simulink model "Overflow"  (R2017b)
settings: Solver=VariableStepAuto  StartTime=0.0  StopTime=10.0  RelTol=1e-3
settings Model: Creator=MrGoshak  LastModifiedBy=MrGoshak

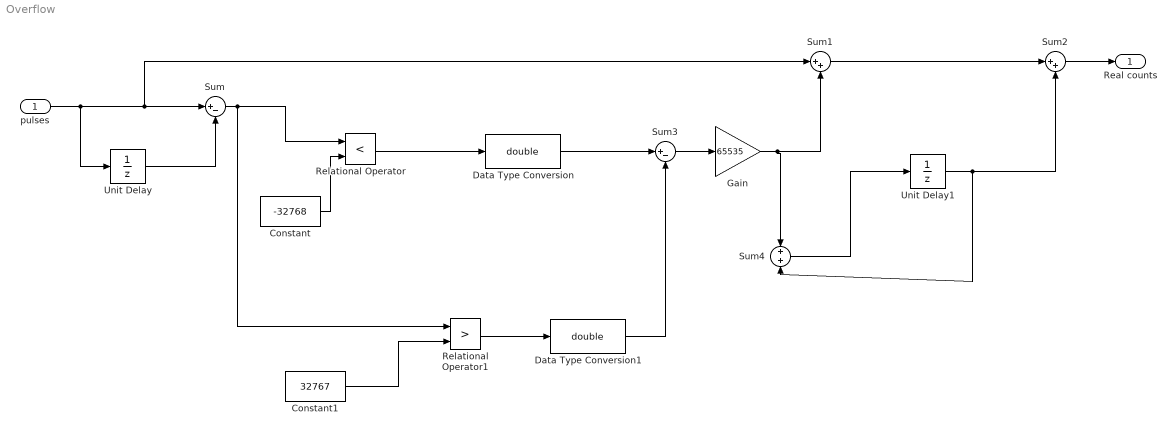
== system Overflow ==
  pulses : Inport
  Constant : Constant  Value=-32768  VectorParams1D=off
  Constant1 : Constant  Value=32767  VectorParams1D=off
  Data Type Conversion : DataTypeConversion  OutDataTypeStr=double
  Data Type Conversion1 : DataTypeConversion  OutDataTypeStr=double
  Gain : Gain  Gain=65535
  Relational Operator : RelationalOperator  Operator=<  OutDataTypeStr=boolean  RndMeth=Simplest
  Relational Operator1 : RelationalOperator  Operator=>  OutDataTypeStr=boolean  RndMeth=Simplest
  Sum : Sum  Inputs=|+-
  Sum1 : Sum  Inputs=|++
  Sum2 : Sum  Inputs=|++
  Sum3 : Sum  Inputs=|+-
  Sum4 : Sum
  Unit Delay : UnitDelay  SampleTime=-1
  Unit Delay1 : UnitDelay  SampleTime=-1
  Real counts : Outport
  wires:
  Unit Delay/1 -> Sum/2
  pulses/1 -> Unit Delay/1, Sum1/1, Sum/1
  Sum1/1 -> Sum2/1
  Sum/1 -> Relational Operator1/1, Relational Operator/1
  Constant/1 -> Relational Operator/2
  Relational Operator/1 -> Data Type Conversion/1
  Data Type Conversion/1 -> Sum3/1
  Constant1/1 -> Relational Operator1/2
  Relational Operator1/1 -> Data Type Conversion1/1
  Data Type Conversion1/1 -> Sum3/2
  Gain/1 -> Sum4/1, Sum1/2
  Sum3/1 -> Gain/1
  Unit Delay1/1 -> Sum4/2, Sum2/2
  Sum4/1 -> Unit Delay1/1
  Sum2/1 -> Real counts/1
